simulink model "quadrotor_strategy_adrc"  (R2026a)
settings: Solver=ode4  StopTime=quad_stop_time  FixedStep=0.02
undefined symbols (not defined in the file): quad_model_id, quad_param_vec, quad_scenario_id, quad_x0
Description:
  | ADRC策略模型：ESO估计总扰动，外环按估计扰动进行主动补偿。
settings Model: Creator=audib  LastModifiedBy=audib

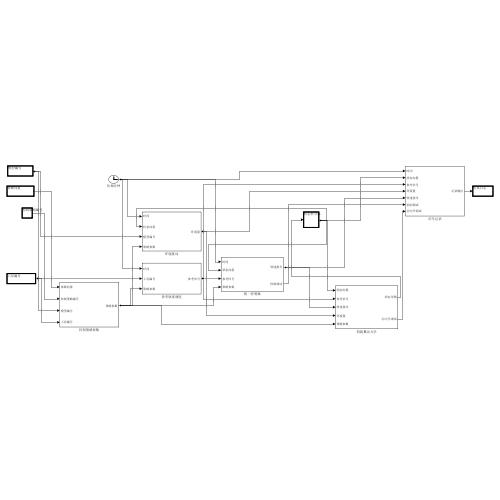
[thumbnail: Simulink's stored preview of the top-level diagram]
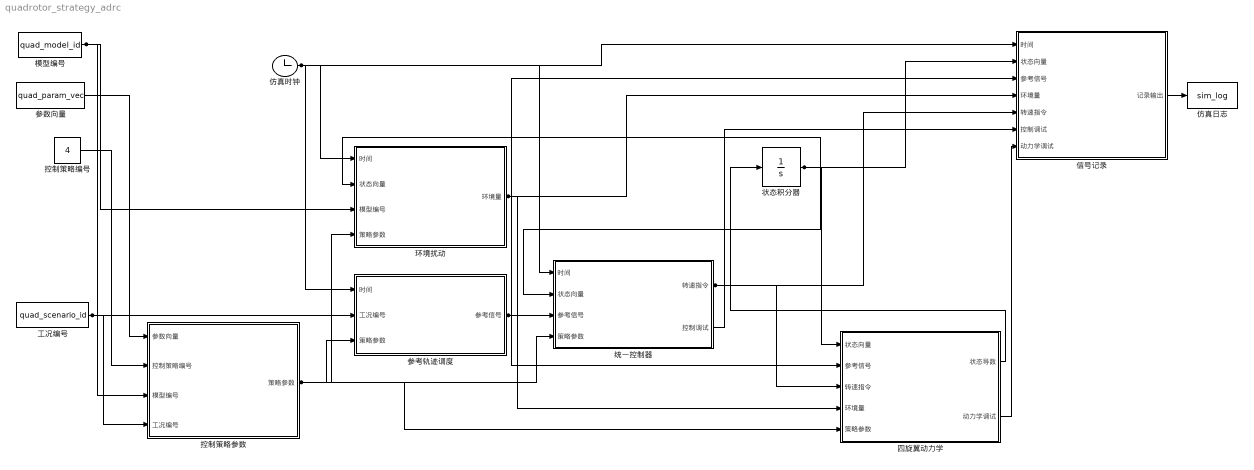
== system quadrotor_strategy_adrc ==
  仿真日志 : ToWorkspace  VariableName=sim_log  SampleTime=-1
  仿真时钟 : Clock
  信号记录 : Subsystem
  参数向量 : Constant  Value=quad_param_vec
  参考轨迹调度 : Subsystem
  四旋翼动力学 : Subsystem
  工况编号 : Constant  Value=quad_scenario_id
  控制策略参数 : Subsystem
  控制策略编号 : Constant  Value=4
  模型编号 : Constant  Value=quad_model_id
  状态积分器 : Integrator  InitialCondition=quad_x0
  环境扰动 : Subsystem
  统一控制器 : Subsystem
  wires:
  模型编号/1 -> 控制策略参数/3(模型编号), 环境扰动/3(模型编号)
  控制策略参数/1(策略参数) -> 四旋翼动力学/5(策略参数), 统一控制器/4(策略参数), 环境扰动/4(策略参数), 参考轨迹调度/3(策略参数)
  控制策略编号/1 -> 控制策略参数/2(控制策略编号)
  工况编号/1 -> 参考轨迹调度/2(工况编号), 控制策略参数/4(工况编号)
  参数向量/1 -> 控制策略参数/1(参数向量)
  仿真时钟/1 -> 信号记录/1(时间), 统一控制器/1(时间), 参考轨迹调度/1(时间), 环境扰动/1(时间)
  环境扰动/1(环境量) -> 四旋翼动力学/4(环境量), 信号记录/4(环境量)
  参考轨迹调度/1(参考信号) -> 四旋翼动力学/2(参考信号), 信号记录/3(参考信号), 统一控制器/3(参考信号)
  统一控制器/1(转速指令) -> 四旋翼动力学/3(转速指令), 信号记录/5(转速指令)
  统一控制器/2(控制调试) -> 信号记录/6(控制调试)
  状态积分器/1 -> 环境扰动/2(状态向量), 信号记录/2(状态向量), 四旋翼动力学/1(状态向量), 统一控制器/2(状态向量)
  四旋翼动力学/1(状态导数) -> 状态积分器/1
  四旋翼动力学/2(动力学调试) -> 信号记录/7(动力学调试)
  信号记录/1(记录输出) -> 仿真日志/1

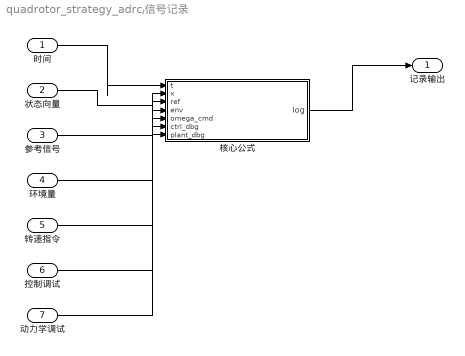
== system quadrotor_strategy_adrc/信号记录 ==
  时间 : Inport
  状态向量 : Inport  Port=2
  参考信号 : Inport  Port=3
  环境量 : Inport  Port=4
  转速指令 : Inport  Port=5
  控制调试 : Inport  Port=6
  动力学调试 : Inport  Port=7
  核心公式 : MATLAB Function  TreatAsAtomicUnit=on
  记录输出 : Outport
  wires:
  时间/1 -> 核心公式/1(t)
  状态向量/1 -> 核心公式/2(x)
  参考信号/1 -> 核心公式/3(ref)
  环境量/1 -> 核心公式/4(env)
  转速指令/1 -> 核心公式/5(omega_cmd)
  控制调试/1 -> 核心公式/6(ctrl_dbg)
  动力学调试/1 -> 核心公式/7(plant_dbg)
  核心公式/1(log) -> 记录输出/1

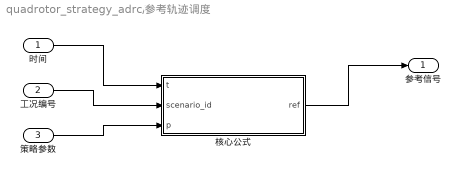
== system quadrotor_strategy_adrc/参考轨迹调度 ==
  时间 : Inport
  工况编号 : Inport  Port=2
  策略参数 : Inport  Port=3
  核心公式 : MATLAB Function  TreatAsAtomicUnit=on
  参考信号 : Outport
  wires:
  时间/1 -> 核心公式/1(t)
  工况编号/1 -> 核心公式/2(scenario_id)
  策略参数/1 -> 核心公式/3(p)
  核心公式/1(ref) -> 参考信号/1

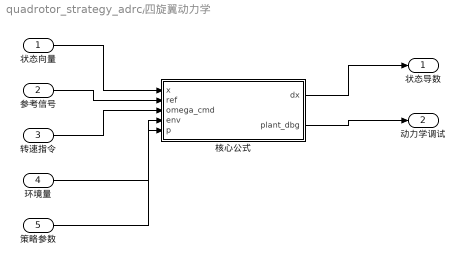
== system quadrotor_strategy_adrc/四旋翼动力学 ==
  状态向量 : Inport
  参考信号 : Inport  Port=2
  转速指令 : Inport  Port=3
  环境量 : Inport  Port=4
  策略参数 : Inport  Port=5
  核心公式 : MATLAB Function  TreatAsAtomicUnit=on
  状态导数 : Outport
  动力学调试 : Outport  Port=2
  wires:
  状态向量/1 -> 核心公式/1(x)
  参考信号/1 -> 核心公式/2(ref)
  转速指令/1 -> 核心公式/3(omega_cmd)
  环境量/1 -> 核心公式/4(env)
  策略参数/1 -> 核心公式/5(p)
  核心公式/1(dx) -> 状态导数/1
  核心公式/2(plant_dbg) -> 动力学调试/1

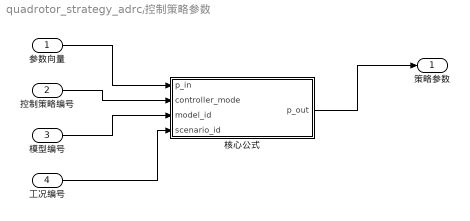
== system quadrotor_strategy_adrc/控制策略参数 ==
  参数向量 : Inport
  控制策略编号 : Inport  Port=2
  模型编号 : Inport  Port=3
  工况编号 : Inport  Port=4
  核心公式 : MATLAB Function  TreatAsAtomicUnit=on
  策略参数 : Outport
  wires:
  参数向量/1 -> 核心公式/1(p_in)
  控制策略编号/1 -> 核心公式/2(controller_mode)
  模型编号/1 -> 核心公式/3(model_id)
  工况编号/1 -> 核心公式/4(scenario_id)
  核心公式/1(p_out) -> 策略参数/1

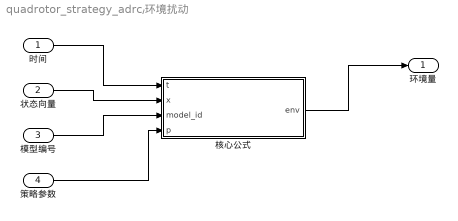
== system quadrotor_strategy_adrc/环境扰动 ==
  时间 : Inport
  状态向量 : Inport  Port=2
  模型编号 : Inport  Port=3
  策略参数 : Inport  Port=4
  核心公式 : MATLAB Function  TreatAsAtomicUnit=on
  环境量 : Outport
  wires:
  时间/1 -> 核心公式/1(t)
  状态向量/1 -> 核心公式/2(x)
  模型编号/1 -> 核心公式/3(model_id)
  策略参数/1 -> 核心公式/4(p)
  核心公式/1(env) -> 环境量/1

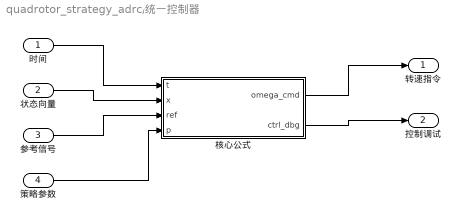
== system quadrotor_strategy_adrc/统一控制器 ==
  时间 : Inport
  状态向量 : Inport  Port=2
  参考信号 : Inport  Port=3
  策略参数 : Inport  Port=4
  核心公式 : MATLAB Function  TreatAsAtomicUnit=on
  转速指令 : Outport
  控制调试 : Outport  Port=2
  wires:
  时间/1 -> 核心公式/1(t)
  状态向量/1 -> 核心公式/2(x)
  参考信号/1 -> 核心公式/3(ref)
  策略参数/1 -> 核心公式/4(p)
  核心公式/1(omega_cmd) -> 转速指令/1
  核心公式/2(ctrl_dbg) -> 控制调试/1

== matlab function quadrotor_strategy_adrc/参考轨迹调度/核心公式 ==
  data: t input; ref output; scenario_id input; p input
function ref = fcn(t, scenario_id, p)
%#codegen
ref = quadrotor_reference_core(t, scenario_id, p);
end

== matlab function quadrotor_strategy_adrc/控制策略参数/核心公式 ==
  data: p_in input; p_out output; controller_mode input; model_id input; scenario_id input
function p_out = fcn(p_in, controller_mode, model_id, scenario_id)
%#codegen
p_out = p_in;
p_out(88) = scenario_id;
p_out(89) = controller_mode;
p_out(90) = model_id;
p_out(97) = 1.0;
end

== matlab function quadrotor_strategy_adrc/环境扰动/核心公式 ==
  data: t input; env output; x input; model_id input; p input
function env = fcn(t, x, model_id, p)
%#codegen
env = quadrotor_environment_core(t, x, model_id, p);
end

== matlab function quadrotor_strategy_adrc/统一控制器/核心公式 ==
  data: t input; omega_cmd output; x input; ref input; p input; ctrl_dbg output
function [omega_cmd, ctrl_dbg] = fcn(t, x, ref, p)
%#codegen
[omega_cmd, ctrl_dbg] = quadrotor_controller_core(t, x, ref, p);
end

== matlab function quadrotor_strategy_adrc/四旋翼动力学/核心公式 ==
  data: x input; dx output; ref input; omega_cmd input; env input; p input; plant_dbg output
function [dx, plant_dbg] = fcn(x, ref, omega_cmd, env, p)
%#codegen
[dx, plant_dbg] = quadrotor_rhs_core(x, ref, omega_cmd, env, p);
end

== matlab function quadrotor_strategy_adrc/信号记录/核心公式 ==
  data: t input; log output; x input; ref input; env input; omega_cmd input; ctrl_dbg input; plant_dbg input
function log = fcn(t, x, ref, env, omega_cmd, ctrl_dbg, plant_dbg)
%#codegen
log = quadrotor_pack_log_core(t, x, ref, env, omega_cmd, ctrl_dbg, plant_dbg);
end
